simulink model "prikaztemp"  (R2015b)
settings: Solver=FixedStepAuto  StartTime=0.0  StopTime=inf  FixedStep=0.001  RelTol=1e-3
undefined symbols (not defined in the file): analoginput
libraries: daqlib x1
settings Model: Creator=ASIJA  LastModifiedBy=ASIJA

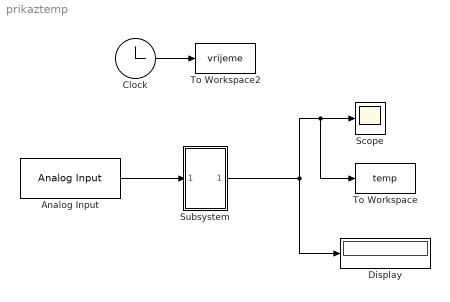
== system prikaztemp ==
  Analog Input : daqlib/Analog Input  AcqMode=0  DeviceMenu=mcc 0 (DEMO-BOARD)  Device=mcc 1 (USB-1208FS)  ObjConstructor=analoginput('mcc',1)  SampleRate=1000  ActualRate=1000  SamplesPerFrame=1  InputType=Differential  NChannelsSelected=1  Channels=0$0$$8$#0$1$$8$#1$2$$8$#0$3$$8$#  NPorts=1 for all hardware channels  DataType=double
      settings: SignalType=Sample-based
  Clock : Clock
  Display : Display
  Scope : Scope
  Subsystem : Subsystem
  To Workspace : ToWorkspace  VariableName=temp  SampleTime=-1
      settings: Save2DSignal=2-D array (concatenate along first dimension)
  To Workspace2 : ToWorkspace  VariableName=vrijeme  SampleTime=-1
      settings: Save2DSignal=2-D array (concatenate along first dimension)
  wires:
  Clock/1 -> To Workspace2/1
  Subsystem/1(Out1) -> To Workspace/1, Scope/1, Display/1
  Analog Input/1 -> Subsystem/1(In1)

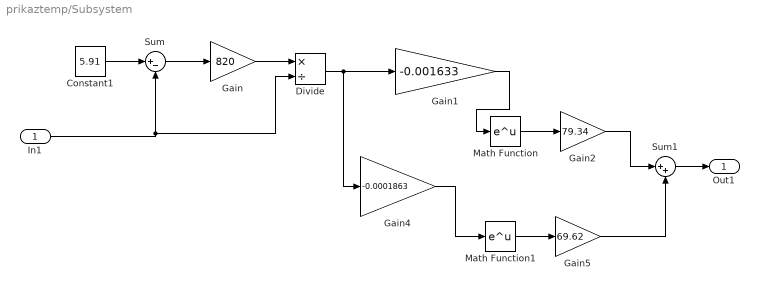
== system prikaztemp/Subsystem ==
  In1 : Inport
  Constant1 : Constant  Value=5.91
  Divide : Product  Inputs=*/
  Gain : Gain  Gain=820
  Gain1 : Gain  Gain=-0.001633
  Gain2 : Gain  Gain=79.34
  Gain4 : Gain  Gain=-0.0001863
  Gain5 : Gain  Gain=69.62
  Math Function : Math  SaturateOnIntegerOverflow=on
  Math Function1 : Math  SaturateOnIntegerOverflow=on
  Sum : Sum  Inputs=|+-
  Sum1 : Sum  Inputs=|++
  Out1 : Outport
  wires:
  Constant1/1 -> Sum/1
  Sum1/1 -> Out1/1
  Math Function/1 -> Gain2/1
  Gain4/1 -> Math Function1/1
  Divide/1 -> Gain4/1, Gain1/1
  Gain1/1 -> Math Function/1
  Gain/1 -> Divide/1
  In1/1 -> Divide/2, Sum/2
  Gain5/1 -> Sum1/2
  Math Function1/1 -> Gain5/1
  Gain2/1 -> Sum1/1
  Sum/1 -> Gain/1
